simulink library "Library_Steering"  (R2023a)
settings: Solver=VariableStepAuto  StartTime=0.0  StopTime=10.0  RelTol=1e-3
undefined symbols (not defined in the file or in its folder): SteeringLeft, SteeringRight
libraries: mbd_s32k1xx_ec_toolbox x17, simulink x8, $bdroot x3
(part 2 of 2)

== stateflow chart Library_Steering/Steering_Mgmt_FSM/Chart ==
  state CAN_Watchdog [parallel]
    entry:
    lastCANWatchDogTime = 0;
    settings: executionOrder=2
    state CAN_Good
    state CAN_Lost
    (default) -> CAN_Good
    CAN_Good -> CAN_Watchdog [order 2] : [input_CAN_timeStamp > lastCANWatchDogTime]{lastCANWatchDogTime = input_CAN_timeStamp}
    CAN_Good -> CAN_Lost [order 1] : [elapsed > param_CANTimeOut & lastCANWatchDogTime ~= 0]{send(CAN_WD_Timeout,Steering_Mode)}
    CAN_Lost -> CAN_Good : FAULT_RESET
  state Steering_Mode [parallel]
    % ALL SDO TRANSFERS MUST BE MADE IN THIS STATE AND NOWHERE ELSE TO AVOID CONFLICTS
    settings: executionOrder=4
    state Steering_Degraded
      entry:
      output_chart_state = 2;
      state SetCaptureMode
        entry:
        output_chart_substate = uint8(hex2dec('21'));
        % Shut off SDO output enable
        output_SDO_enable = 0;
        exit:
        % Shut off SDO output upon exiting this state
        output_SDO_enable = 0;
        state SDOSend
          entry:
          output_SDO_enable = 0;
          output_SDO_data = cast([hex2dec('2B'); hex2dec('00'); hex2dec('24'); 0; hex2dec('45'); hex2dec('05'); 0; 0;],'uint8');
          output_SDO_enable = 1;
        state SDOWait1
          entry:
          output_SDO_enable = 0;
          output_SDO_data = cast([hex2dec('40'); hex2dec('00'); hex2dec('24'); 0; 0; 0; 0; 0],'uint8');
          output_SDO_enable = 1;
        state SDOWait2
          entry:
          output_SDO_enable = 0;
        (default) -> Steering_Mode.Steering_Degraded.SetCaptureMode.SDOSend
        Steering_Mode.Steering_Degraded.SetCaptureMode.SDOSend -> Steering_Mode.Steering_Degraded.SetCaptureMode.SDOWait1 : [input_SDOBuffer == 0]
        Steering_Mode.Steering_Degraded.SetCaptureMode.SDOWait2 -> Steering_Mode.Steering_Degraded.SetCaptureMode.SDOSend : [elapsed > 0.5 && input_SDOBuffer == 0]
        Steering_Mode.Steering_Degraded.SetCaptureMode.SDOWait1 -> Steering_Mode.Steering_Degraded.SetCaptureMode.SDOWait2 : [input_SDOBuffer == 0]
      state SetVelocityLimit
        entry:
        output_chart_substate = uint8(hex2dec('22'));
        % Shut off SDO output enable
        output_SDO_enable = 0;
        exit:
        % Shut off SDO output upon exiting this state
        output_SDO_enable = 0;
        state SDOSend
          entry:
          output_SDO_enable = 0;
          output_SDO_data = cast([hex2dec('23'); hex2dec('80'); hex2dec('60'); 0; 32; 3; 0; 0;],'uint8');
          output_SDO_enable = 1;
        state SDOWait1
          entry:
          output_SDO_enable = 0;
          output_SDO_data = cast([hex2dec('40'); hex2dec('80'); hex2dec('60'); 0; 0; 0; 0; 0],'uint8');
          output_SDO_enable = 1;
        state SDOWait2
          entry:
          output_SDO_enable = 0;
        (default) -> Steering_Mode.Steering_Degraded.SetVelocityLimit.SDOSend
        Steering_Mode.Steering_Degraded.SetVelocityLimit.SDOSend -> Steering_Mode.Steering_Degraded.SetVelocityLimit.SDOWait1 : [input_SDOBuffer == 0]
        Steering_Mode.Steering_Degraded.SetVelocityLimit.SDOWait2 -> Steering_Mode.Steering_Degraded.SetVelocityLimit.SDOSend : [elapsed > 0.5 && input_SDOBuffer == 0]
        Steering_Mode.Steering_Degraded.SetVelocityLimit.SDOWait1 -> Steering_Mode.Steering_Degraded.SetVelocityLimit.SDOWait2 : [input_SDOBuffer == 0]
      state SetCSPMode
        entry:
        output_chart_substate = uint8(hex2dec('23'));
        % Shut off SDO output enable
        output_SDO_enable = 0;
        exit:
        % Shut off SDO output upon exiting this state
        output_SDO_enable = 0;
        state SDOSend
          entry:
          output_SDO_enable = 0;
          output_SDO_data = cast([hex2dec('2F'); hex2dec('60'); hex2dec('60'); 0; 8; 0; 0; 0;],'uint8');
          output_SDO_enable = 1;
        state SDOWait1
          entry:
          output_SDO_enable = 0;
          output_SDO_data = cast([hex2dec('40'); hex2dec('60'); hex2dec('60'); 0; 0; 0; 0; 0],'uint8');
          output_SDO_enable = 1;
        state SDOWait2
          entry:
          output_SDO_enable = 0;
        (default) -> Steering_Mode.Steering_Degraded.SetCSPMode.SDOSend
        Steering_Mode.Steering_Degraded.SetCSPMode.SDOSend -> Steering_Mode.Steering_Degraded.SetCSPMode.SDOWait1 : [input_SDOBuffer == 0]
        Steering_Mode.Steering_Degraded.SetCSPMode.SDOWait2 -> Steering_Mode.Steering_Degraded.SetCSPMode.SDOSend : [elapsed > 0.5 && input_SDOBuffer == 0]
        Steering_Mode.Steering_Degraded.SetCSPMode.SDOWait1 -> Steering_Mode.Steering_Degraded.SetCSPMode.SDOWait2 : [input_SDOBuffer == 0]
      state CheckForCaptures
        entry:
        output_chart_substate = uint8(hex2dec('24'));
        % Shut off SDO output enable
        output_SDO_enable = 0;
        % Enable transmission for the position target PDO
        output_PDO_enable = 1;
        exit:
        output_SDO_enable = 0;
        state SDOSend
          entry:
          output_SDO_enable = 0;
          output_SDO_data = cast([hex2dec('40'); hex2dec('01'); hex2dec('24'); 0; 0; 0; 0; 0;],'uint8');
          output_SDO_enable = 1;
        state SDOWait2
          entry:
          output_SDO_enable = 0;
        (default) -> Steering_Mode.Steering_Degraded.CheckForCaptures.SDOSend
        Steering_Mode.Steering_Degraded.CheckForCaptures.SDOSend -> Steering_Mode.Steering_Degraded.CheckForCaptures.SDOWait2
        Steering_Mode.Steering_Degraded.CheckForCaptures.SDOWait2 -> Steering_Mode.Steering_Degraded.CheckForCaptures.SDOSend : [input_SDOBuffer == 0]
      state FinalCalibration
        output_chart_substate = uint8(hex2dec('25'));
        % Shut off SDO output enable
        output_SDO_enable = 0;
        % Keep the PDO enabled for the position setpoint update
        output_PDO_enable = 1;
        exit:
        % Shut off SDO output upon exiting this state
        output_SDO_enable = 0;
        output_PDO_enable = 1;
        state RequestIndexPos
          entry:
          output_SDO_enable = 0;
          output_SDO_data = cast([hex2dec('40'); hex2dec('02'); hex2dec('24'); 0; 0; 0; 0; 0;],'uint8');
          output_SDO_enable = 1;
        state RequestHomePos
          entry:
          output_SDO_enable = 0;
          output_SDO_data = cast([hex2dec('40'); hex2dec('03'); hex2dec('24'); 0; 0; 0; 0; 0;],'uint8');
          output_SDO_enable = 1;
        state RequestHighSpeedCapturePos
          entry:
          output_SDO_enable = 0;
          output_SDO_data = cast([hex2dec('40'); hex2dec('05'); hex2dec('24'); 0; 0; 0; 0; 0;],'uint8');
          output_SDO_enable = 1;
        state WaitForIndexPos
          entry:
          output_SDO_enable = 0;
        state WaitForHomePos1
          entry:
          output_SDO_enable = 0;
        state WaitForHighSpeedCapturePos
          entry:
          output_SDO_enable = 0;
        state StoreIndex
          entry:
          output_SDO_enable = 0;
          index_position = SDO2Integer32(input_SDO_message);
        state StoreHome
          entry:
          output_SDO_enable = 0;
          home_position = SDO2Integer32(input_SDO_message);
        state StoreHighSpeedCapturePos
          entry:
          output_SDO_enable = 0;
          highspeed_position = SDO2Integer32(input_SDO_message);
        state CalculateZeroOffset
          entry:
          output_SDO_enable = 0;
          hall_width = highspeed_position - home_position;
          int_offset_2 = floor((highspeed_position - index_position)/(4000));
          int_offset_1 = floor((home_position - index_position)/(4000));
          home_index = index_position + 4000*max(int_offset_1,int_offset_2);
          home_offset = min(home_position - home_index,highspeed_position - home_index);
          final_offset = home_index;
        (default) -> RequestIndexPos
        StoreIndex -> RequestHomePos : [input_SDOBuffer == 0]
        StoreHome -> RequestHighSpeedCapturePos : [input_SDOBuffer == 0]
        RequestIndexPos -> WaitForIndexPos : [input_SDOBuffer == 0]
        WaitForIndexPos -> RequestIndexPos [order 2] : [elapsed > 0.5 && input_SDOBuffer == 0]
        RequestHomePos -> WaitForHomePos1 : [input_SDOBuffer == 0]
        WaitForHomePos1 -> RequestHomePos [order 2] : [elapsed > 0.5 && input_SDOBuffer == 0]
        RequestHighSpeedCapturePos -> WaitForHighSpeedCapturePos : [input_SDOBuffer == 0]
        WaitForHighSpeedCapturePos -> RequestHighSpeedCapturePos [order 2] : [elapsed > 0.5 && input_SDOBuffer == 0]
        WaitForIndexPos -> StoreIndex [order 1] : [input_SDO_message(2) == hex2dec('02') && input_SDO_message(3) == hex2dec('24')]
        WaitForHomePos1 -> StoreHome [order 1] : [input_SDO_message(2) == hex2dec('03') && input_SDO_message(3) == hex2dec('24')]
        WaitForHighSpeedCapturePos -> StoreHighSpeedCapturePos [order 1] : [input_SDO_message(2) == hex2dec('05') && input_SDO_message(3) == hex2dec('24')]
        StoreHighSpeedCapturePos -> CalculateZeroOffset
      state SetOffset
        % Set Index 0x607C with a new value to adjust the zero position of the steering system relative to the arbitary home that was set at startup
        entry:
        final_offset = final_offset + param_finalOffsetAlignment;
        output_chart_substate = uint8(hex2dec('26'));
        output_PDO_enable = 1;
        output_position_offset = 0;
        offset_bytes = [0; 0; 0; 0];
        offset_bytes(1) = extractByte(output_position_offset,1);
        offset_bytes(2) = extractByte(output_position_offset,2);
        offset_bytes(3) = extractByte(output_position_offset,3);
        offset_bytes(4) = extractByte(output_position_offset,4);
        state SDOSend
          entry:
          offset_bytes(1) = extractByte(output_position_offset,1);
          offset_bytes(2) = extractByte(output_position_offset,2);
          offset_bytes(3) = extractByte(output_position_offset,3);
          offset_bytes(4) = extractByte(output_position_offset,4);
          output_SDO_enable = 0;
          output_SDO_data = cast([hex2dec('23'); hex2dec('B0'); hex2dec('60'); 0; offset_bytes],'uint8');
          output_SDO_enable = 1;
        state SDOWait1
          entry:
          output_SDO_enable = 0;
          output_SDO_data = cast([hex2dec('40'); hex2dec('B0'); hex2dec('60'); 0; 0; 0; 0; 0],'uint8');
          output_SDO_enable = 1;
        state SDOWait2
          entry:
          output_SDO_enable = 0;
        (default) -> Steering_Mode.Steering_Degraded.SetOffset.SDOSend
        Steering_Mode.Steering_Degraded.SetOffset.SDOWait2 -> Steering_Mode.Steering_Degraded.SetOffset.SDOSend : [elapsed > 0.02 && input_SDOBuffer == 0]{output_position_offset = sign(final_offset)*min(abs(output_position_offset)+...
            | param_alignmentSlewRate,abs(final_offset));}
        Steering_Mode.Steering_Degraded.SetOffset.SDOSend -> Steering_Mode.Steering_Degraded.SetOffset.SDOWait1 : [input_SDOBuffer == 0]
        Steering_Mode.Steering_Degraded.SetOffset.SDOWait1 -> Steering_Mode.Steering_Degraded.SetOffset.SDOWait2 : [all(input_SDO_message(2:8) == cast([hex2dec('B0');...
            |  hex2dec('60'); 0; offset_bytes],'uint8'))]
      state SetVelocityLimit1
        entry:
        output_chart_substate = uint8(hex2dec('27'));
        % Shut off SDO output enable
        output_SDO_enable = 0;
        exit:
        % Shut off SDO output upon exiting this state
        output_SDO_enable = 0;
        state SDOSend
          entry:
          output_SDO_enable = 0;
          output_SDO_data = cast([hex2dec('23'); hex2dec('80'); hex2dec('60'); 0; 255; 79; 0; 0;],'uint8');
          output_SDO_enable = 1;
        state SDOWait1
          entry:
          output_SDO_enable = 0;
          output_SDO_data = cast([hex2dec('40'); hex2dec('80'); hex2dec('60'); 0; 0; 0; 0; 0],'uint8');
          output_SDO_enable = 1;
        state SDOWait2
          entry:
          output_SDO_enable = 0;
        (default) -> Steering_Mode.Steering_Degraded.SetVelocityLimit1.SDOSend
        Steering_Mode.Steering_Degraded.SetVelocityLimit1.SDOSend -> Steering_Mode.Steering_Degraded.SetVelocityLimit1.SDOWait1 : [input_SDOBuffer == 0]
        Steering_Mode.Steering_Degraded.SetVelocityLimit1.SDOWait2 -> Steering_Mode.Steering_Degraded.SetVelocityLimit1.SDOSend : [elapsed > 0.5 && input_SDOBuffer == 0]
        Steering_Mode.Steering_Degraded.SetVelocityLimit1.SDOWait1 -> Steering_Mode.Steering_Degraded.SetVelocityLimit1.SDOWait2 : [input_SDOBuffer == 0]
      (default) -> SetCaptureMode
      SetCaptureMode -> SetVelocityLimit : [all(input_SDO_message == cast([hex2dec('4B'); hex2dec('00'); hex2dec('24'); 0; hex2dec('45'); hex2dec('05'); 0; 0;],'uint8'))]
      SetVelocityLimit -> SetCSPMode : [all(input_SDO_message == cast([hex2dec('43'); hex2dec('80'); hex2dec('60'); 0; 32; 3; 0; 0;],'uint8'))]
      SetCSPMode -> CheckForCaptures : [all(input_SDO_message == cast([hex2dec('4F'); hex2dec('60'); hex2dec('60'); 0; 8; 0; 0; 0;],'uint8'))]
      CalculateZeroOffset -> CheckForCaptures [order 2]
      CheckForCaptures -> FinalCalibration : [input_SDO_message(2) == hex2dec('01') &&...
          |  input_SDO_message(3) == hex2dec('24') &&...
          |  bitand(uint8(hex2dec('11')),input_SDO_message(5)) == uint8(hex2dec('11')) &&...
          |  bitand(uint8(hex2dec('01')),input_SDO_message(6)) == uint8(hex2dec('01'))]
      CalculateZeroOffset -> SetOffset [order 1] : [final_offset < param_finalOffsetHighThresh && final_offset > param_finalOffsetLowThresh && ...
          | [hall_width > param_hallWidthLowThresh && hall_width < param_hallWidthHighThresh && ...
          | home_offset > param_homeOffsetLowThresh && home_offset < param_homeOffsetHighThresh && ...
          | int_offset_1 - int_offset_2 < param_intOffsetThresh && int_offset_2 - int_offset_1 < param_intOffsetThresh]]
      SetOffset -> SetVelocityLimit1 : [output_position_offset == final_offset]
    state Steering_Operational
      entry:
      output_chart_state = 3
      output_chart_substate = uint8(hex2dec('30'));
      output_PDO_enable = 1;
      output_SDO_data = cast([hex2dec('40');...
      hex2dec('41'); hex2dec('60'); hex2dec('00');...
      hex2dec('00'); hex2dec('00'); hex2dec('00');...
      hex2dec('00')],'uint8');
      output_SDO_enable = 1;
      output_actual_position = SDO2Integer32(input_SDO_message);
    state Steering_Startup
      entry:
      output_chart_state = 1;
      state ConfirmNMTUp  % Sends NMT (network management) message to start up the CANOpen node being controlled
        % Actions to perform once upon entering this state
        entry:
        % Set chart state indicator variable
        output_chart_substate = uint8(hex2dec('11'));
        % Actions to perform once when exiting this state
        exit:
        % Disable the NMT message send output port when done
        output_NMT_enable = 0;
        output_SDO_enable = 0;
        state NMTQuerySend  % Send the NMT query message via SDO format
          entry:
          % Set the SDO data packet to request the device network status word (0x21B4)
          output_SDO_data = cast([hex2dec('40'); hex2dec('B4'); ...
          hex2dec('21'); hex2dec('00'); hex2dec('00');...
          hex2dec('00'); hex2dec('00'); hex2dec('00')],'uint8');
          % Enable the SDO send
          output_SDO_enable = 1;
        state SDOWait  % Wait to send next SDO message
          entry:
          output_NMT_enable = 0;
        state NMTSetActive % Enable the block that sends the NMT active message
          entry:
          % Enable the NMT send
          output_NMT_enable = 1;
        state NMTWait  % Wait to send next NMT message
          entry:
          output_SDO_enable = 0;
        (default) -> Steering_Mode.Steering_Startup.ConfirmNMTUp.SDOWait  % Wait to send next SDO message
        Steering_Mode.Steering_Startup.ConfirmNMTUp.SDOWait  % Wait to send next SDO message -> Steering_Mode.Steering_Startup.ConfirmNMTUp.NMTQuerySend  % Send the NMT query message via SDO format : [input_SDOBuffer == 0]
        Steering_Mode.Steering_Startup.ConfirmNMTUp.NMTSetActive % Enable the block that sends the NMT active message -> Steering_Mode.Steering_Startup.ConfirmNMTUp.SDOWait  % Wait to send next SDO message
        Steering_Mode.Steering_Startup.ConfirmNMTUp.NMTQuerySend  % Send the NMT query message via SDO format -> Steering_Mode.Steering_Startup.ConfirmNMTUp.NMTWait  % Wait to send next NMT message
        Steering_Mode.Steering_Startup.ConfirmNMTUp.NMTWait  % Wait to send next NMT message -> Steering_Mode.Steering_Startup.ConfirmNMTUp.NMTSetActive % Enable the block that sends the NMT active message : [input_NMTBuffer == 0]
      state CheckEnableAmpStatus  % Sends SDO message until the amp status message shows that it is enabled
        % Actions to perform once upon entering this state
        entry:
        % Set chart state indicator variable
        output_chart_substate = uint8(hex2dec('12'));
        state StatusQuerySend  % Send the amp status query message via SDO format
          entry:
          % Set the SDO data packet to request the amp status word (0x6041)
          output_SDO_data = cast([hex2dec('40'); hex2dec('41'); ...
          hex2dec('60'); hex2dec('00'); hex2dec('00');...
          hex2dec('00'); hex2dec('00'); hex2dec('00')],'uint8');
          % Enable the SDO send
          output_SDO_enable = 1;
        state SDOWait  % Wait to send next SDO message
          entry:
          output_SDO_enable = 0;
        state SetAmpEnabled % Enable the block that sends the amp enable message
          entry:
          % Set the SDO data packet to set the amp control word (0x6040)
          output_SDO_data = cast([hex2dec('2B'); hex2dec('40'); ...
          hex2dec('60'); hex2dec('00'); hex2dec('07');...
          hex2dec('00'); hex2dec('00'); hex2dec('00')],'uint8');
          % Enable the SDO send
          output_SDO_enable = 1;
        state SDOWait1  % Wait to send next NMT message
          entry:
          output_SDO_enable = 0;
        (default) -> Steering_Mode.Steering_Startup.CheckEnableAmpStatus.SDOWait  % Wait to send next SDO message
        Steering_Mode.Steering_Startup.CheckEnableAmpStatus.SDOWait  % Wait to send next SDO message -> Steering_Mode.Steering_Startup.CheckEnableAmpStatus.StatusQuerySend  % Send the amp status query message via SDO format : [input_SDOBuffer == 0]
        Steering_Mode.Steering_Startup.CheckEnableAmpStatus.SetAmpEnabled % Enable the block that sends the amp enable message -> Steering_Mode.Steering_Startup.CheckEnableAmpStatus.SDOWait  % Wait to send next SDO message
        Steering_Mode.Steering_Startup.CheckEnableAmpStatus.StatusQuerySend  % Send the amp status query message via SDO format -> Steering_Mode.Steering_Startup.CheckEnableAmpStatus.SDOWait1  % Wait to send next NMT message
        Steering_Mode.Steering_Startup.CheckEnableAmpStatus.SDOWait1  % Wait to send next NMT message -> Steering_Mode.Steering_Startup.CheckEnableAmpStatus.SetAmpEnabled % Enable the block that sends the amp enable message : [input_SDOBuffer == 0]
      state CheckOperatingMode  % Sends SDO message until the operating mode is determined, and sends the state machine either to finish startup or resuming operation
        % Actions to perform once upon entering this state
        entry:
        % Set chart state indicator variable
        output_chart_substate = uint8(hex2dec('13'));
        state SDOWait1  % Wait to send next SDO message
          entry:
          output_SDO_enable = 0;
        state ModeQuerySend  % Send the amp status query message via SDO format
          entry:
          % Set the SDO data packet to request the amp status word (0x6041)
          output_SDO_data = cast([hex2dec('40'); hex2dec('61'); ...
          hex2dec('60'); hex2dec('00'); hex2dec('00');...
          hex2dec('00'); hex2dec('00'); hex2dec('00')],'uint8');
          % Enable the SDO send
          output_SDO_enable = 1;
        (default) -> SDOWait1  % Wait to send next SDO message
        SDOWait1  % Wait to send next SDO message -> ModeQuerySend  % Send the amp status query message via SDO format : [input_SDOBuffer == 0]
        ModeQuerySend  % Send the amp status query message via SDO format -> SDOWait1  % Wait to send next SDO message
      state CollectAnalogValues  % Controls acquisition of desired number of analog measurements until an average can be generated
        % Actions to perform once upon entering this state
        entry:
        % Set chart state indicator variable to 0x14
        output_chart_substate = uint8(hex2dec('14'));
        % Initialize a counter for the number of measurements collected
        meas_counter = 0;
        % Initialize a running sum variable to zero
        running_mean = 0;
        % Initialize the running standard deviation variable to zero
        running_std = 0;
        % Initialize a variable to keep track of the time stamp of the most recent SDO message received
        % to avoid duplicating measurements in the average
        prevTime = input_CAN_timeStamp;
        % Set the SDO transmit message to request the analog measurement object
        output_SDO_data = cast([hex2dec('40'); hex2dec('00'); hex2dec('22'); hex2dec('00'); hex2dec('00');...
        hex2dec('00'); hex2dec('00'); hex2dec('00')],'uint8');
        % Enable SDO output transmission (holding this high will send continuously)
        output_SDO_enable = 1;
        % Actions to perform once per cycle
        during:
        % Check for a new SDO message with the analog measurement value. If a new measurement is available, average it
        receiveAnalogInput;
        % Exit condition is that 50 measurements have been averaged together
      state receiveAnalogInput [function]
        (default) -> (junction 364) : {potVoltage = SDO2Integer16(input_SDO_message)}
        (junction 364) -> (junction 365) [order 1] : [potVoltage > param_minPotAvgVal && potVoltage < param_maxPotAvgVal && meas_counter <= param_initNumPotReadings &&...
            |  input_CAN_timeStamp ~= prevTime && input_SDO_message(2) == hex2dec('00') && input_SDO_message(3) == hex2dec('22')]
        (junction 364) -> (junction 366) [order 2]
        (junction 365) -> (junction 367) : {meas_counter = meas_counter + 1;
            |  residual = (cast(potVoltage,'double') - running_mean);
            |  running_mean = running_mean + residual/meas_counter;
            |  running_std = running_std + (residual*(cast(potVoltage,'double') - running_mean) - running_std)/meas_counter;
            |  prevTime = input_CAN_timeStamp;}
        (junction 367) -> (junction 366)
      state WriteHomePos  % Convert the raw analog values to encoder counts and set the motor position object on the amp
        % Actions to perform once upon entering this state
        entry:
        % Set chart state indicator variable to 0x15
        output_chart_substate = uint8(hex2dec('15'));
        % Disable transmission of the SDO message until the message data bytes are updated
        output_SDO_enable = 0;
        % Convert the potentiometer position to encoder counts
        output_actual_position = cast(param_potEncSlope*running_mean + param_potEncInt,'int32');
        pos_encoder_bytes = [0; 0; 0; 0];
        pos_encoder_bytes(1) = extractByte(output_actual_position,1);
        pos_encoder_bytes(2) = extractByte(output_actual_position,2);
        pos_encoder_bytes(3) = extractByte(output_actual_position,3);
        pos_encoder_bytes(4) = extractByte(output_actual_position,4);
        % Set the SDO message data that should be echoed back to move to the next state
        Position_Written_Expected_Bytes = [hex2dec('43'); hex2dec('63'); hex2dec('60'); hex2dec('00'); pos_encoder_bytes];
        exit:
        % Shut off SDO output upon exiting this state
        output_SDO_enable = 0;
        state SDOSend
          entry:
          output_SDO_enable = 0;
          output_SDO_data = cast([hex2dec('23'); hex2dec('63'); hex2dec('60'); hex2dec('00'); pos_encoder_bytes],'uint8');
          output_SDO_enable = 1;
        state SDOWait1
          entry:
          output_SDO_enable = 0;
          output_SDO_data = cast([hex2dec('40'); hex2dec('63'); hex2dec('60'); 0; 0; 0; 0; 0],'uint8');
          output_SDO_enable = 1;
        state SDOWait2
          entry:
          output_SDO_enable = 0;
        (default) -> Steering_Mode.Steering_Startup.WriteHomePos.SDOSend
        Steering_Mode.Steering_Startup.WriteHomePos.SDOSend -> Steering_Mode.Steering_Startup.WriteHomePos.SDOWait1 : [input_SDOBuffer == 0]
        Steering_Mode.Steering_Startup.WriteHomePos.SDOWait2 -> Steering_Mode.Steering_Startup.WriteHomePos.SDOSend : [elapsed > 0.5 && input_SDOBuffer == 0]
        Steering_Mode.Steering_Startup.WriteHomePos.SDOWait1 -> Steering_Mode.Steering_Startup.WriteHomePos.SDOWait2 : [input_SDOBuffer == 0]
      (default) -> Steering_Mode.Steering_Startup.ConfirmNMTUp  % Sends NMT (network management) message to start up the CANOpen node being controlled
      Steering_Mode.Steering_Startup.ConfirmNMTUp  % Sends NMT (network management) message to start up the CANOpen node being controlled -> Steering_Mode.Steering_Startup.CheckEnableAmpStatus  % Sends SDO message until the amp status message shows that it is enabled : [input_SDO_message(2) == cast(hex2dec('B4'),'uint8') && input_SDO_message(3) == cast(hex2dec('21'),'uint8') && bitand(input_SDO_message(5),cast(hex2dec('03'),'uint8')) == cast(3,'uint8')]
      Steering_Mode.Steering_Startup.CheckEnableAmpStatus  % Sends SDO message until the amp status message shows that it is enabled -> CheckOperatingMode  % Sends SDO message until the operating mode is determined, and sends the state machine either to finish startup or resuming operation : [input_SDO_message(2) == cast(hex2dec('41'),'uint8') && input_SDO_message(3) == cast(hex2dec('60'),'uint8') && bitand(input_SDO_message(5),cast(hex2dec('33'),'uint8')) == cast(hex2dec('33'),'uint8')]
      CheckOperatingMode  % Sends SDO message until the operating mode is determined, and sends the state machine either to finish startup or resuming operation -> CollectAnalogValues  % Controls acquisition of desired number of analog measurements until an average can be generated [order 2] : [input_SDO_message(2) == cast(hex2dec('61'),'uint8') && input_SDO_message(3) == cast(hex2dec('60'),'uint8')]
      CollectAnalogValues  % Controls acquisition of desired number of analog measurements until an average can be generated -> (junction 613) : [meas_counter >...
          |  param_initNumPotReadings]
      (junction 613) -> CollectAnalogValues  % Controls acquisition of desired number of analog measurements until an average can be generated [order 2]
      (junction 613) -> WriteHomePos  % Convert the raw analog values to encoder counts and set the motor position object on the amp [order 1] : [running_mean > param_minPotAvgVal && running_mean < param_maxPotAvgVal && running_std < param_maxPotSTD]
    state Steering_Fault
      entry:
      output_chart_substate = uint8(hex2dec('00'));
      output_PDO_enable = 0;
      output_chart_state = 0;
      output_SDO_data = cast([hex2dec('2B');...
      hex2dec('40'); hex2dec('60'); hex2dec('00');...
      hex2dec('05'); hex2dec('00'); hex2dec('00');...
      hex2dec('00')],'uint8');
      output_SDO_enable = 1;
    Steering_Degraded -> Steering_Fault [commented out] : AMP_FAULT
    Steering_Degraded -> Steering_Fault : CAN_WD_Timeout
    Steering_Operational -> Steering_Fault [commented out] : AMP_FAULT
    Steering_Operational -> Steering_Fault : CAN_WD_Timeout
    (default) -> Steering_Startup
    Steering_Startup -> Steering_Fault [order 1] : CAN_WD_Timeout
    Steering_Startup -> Steering_Fault [commented out] : AMP_FAULT
    Steering_Startup -> Steering_Fault [order 2] : [elapsed > param_startupTimeOut]...
        | {startup_timeout = 10}
    Steering_Fault -> Steering_Startup : FAULT_RESET
    CheckOperatingMode  % Sends SDO message until the operating mode is determined, and sends the state machine either to finish startup or resuming operation -> Steering_Degraded [order 1] : [input_SDO_message(2) == cast(hex2dec('61'),'uint8')...
        |  && input_SDO_message(3) == cast(hex2dec('60'),'uint8')...
        |  && input_SDO_message(5) == uint8(8)]
    SetVelocityLimit1 -> Steering_Operational : [all(input_SDO_message == cast([hex2dec('43'); hex2dec('80'); hex2dec('60'); 0; 255; 79; 0; 0;],'uint8'))]
    WriteHomePos  % Convert the raw analog values to encoder counts and set the motor position object on the amp -> Steering_Degraded : [all(input_SDO_message == Position_Written_Expected_Bytes)]
  state Fault_Lamp_Control [parallel]
    settings: executionOrder=1
    state Steady_OFF
      during:
      output_fault_lamp = 0;
    state Blink_OFF
      during:
      output_fault_lamp = 0;
    state Blink_ON
      during:
      output_fault_lamp = 1;
    state Steady_ON
      during:
      output_fault_lamp = 1;
    Steady_OFF -> Fault_Lamp_Control : [output_chart_state ~= 3]
    (junction 517) -> Steady_OFF [order 2] : [output_chart_state == 3]
    Blink_ON -> Steady_OFF [order 1] : [output_chart_state == 3]
    Blink_OFF -> Steady_OFF [order 1] : [output_chart_state == 3]
    Blink_OFF -> Blink_ON [order 3] : [elapsed > output_chart_state*0.2]
    (default) -> (junction 517)
    (junction 517) -> Blink_ON [order 3]
    (junction 517) -> Steady_ON [order 1] : [output_chart_state == 0]
    Blink_ON -> Blink_OFF [order 3] : [elapsed > output_chart_state*0.2]
    Blink_ON -> Steady_ON [order 2] : [output_chart_state == 0]
    Blink_OFF -> Steady_ON [order 2] : [output_chart_state == 0]
    Steady_ON -> Fault_Lamp_Control : [output_chart_state ~= 0]
  state Steering_Fault_Detection [parallel]
    settings: executionOrder=3
    state No_Fault
    state Faulted
      entry:
      send(AMP_FAULT,Steering_Mode)
      state ConfirmNMTUp  % Sends NMT (network management) message to start up the CANOpen node being controlled
        % Actions to perform once upon entering this state
        entry:
        % Set chart state indicator variable
        output_chart_substate = uint8(hex2dec('11'));
        % Actions to perform once when exiting this state
        exit:
        % Disable the NMT message send output port when done
        output_NMT_enable = 0;
        output_SDO_enable = 0;
        state NMTQuerySend  % Send the NMT query message via SDO format
          entry:
          % Set the SDO data packet to request the device network status word (0x21B4)
          output_SDO_data = cast([hex2dec('40'); hex2dec('B4'); ...
          hex2dec('21'); hex2dec('00'); hex2dec('00');...
          hex2dec('00'); hex2dec('00'); hex2dec('00')],'uint8');
          % Enable the SDO send
          output_SDO_enable = 1;
        state SDOWait  % Wait to send next SDO message
          entry:
          output_NMT_enable = 0;
        state NMTSetActive % Enable the block that sends the NMT active message
          entry:
          % Enable the NMT send
          output_NMT_enable = 1;
        state NMTWait  % Wait to send next NMT message
          entry:
          output_SDO_enable = 0;
        (default) -> Steering_Fault_Detection.Faulted.ConfirmNMTUp.SDOWait  % Wait to send next SDO message
        Steering_Fault_Detection.Faulted.ConfirmNMTUp.SDOWait  % Wait to send next SDO message -> Steering_Fault_Detection.Faulted.ConfirmNMTUp.NMTQuerySend  % Send the NMT query message via SDO format : [input_SDOBuffer == 0]
        Steering_Fault_Detection.Faulted.ConfirmNMTUp.NMTSetActive % Enable the block that sends the NMT active message -> Steering_Fault_Detection.Faulted.ConfirmNMTUp.SDOWait  % Wait to send next SDO message
        Steering_Fault_Detection.Faulted.ConfirmNMTUp.NMTQuerySend  % Send the NMT query message via SDO format -> Steering_Fault_Detection.Faulted.ConfirmNMTUp.NMTWait  % Wait to send next NMT message
        Steering_Fault_Detection.Faulted.ConfirmNMTUp.NMTWait  % Wait to send next NMT message -> Steering_Fault_Detection.Faulted.ConfirmNMTUp.NMTSetActive % Enable the block that sends the NMT active message : [input_NMTBuffer == 0]
      state CheckEnableAmpStatus  % Sends SDO message until the amp status message shows that it is enabled
        % Actions to perform once upon entering this state
        entry:
        % Set chart state indicator variable
        output_chart_substate = uint8(hex2dec('12'));
        state StatusQuerySend  % Send the amp status query message via SDO format
          entry:
          % Set the SDO data packet to request the amp status word (0x6041)
          output_SDO_data = cast([hex2dec('40'); hex2dec('41'); ...
          hex2dec('60'); hex2dec('00'); hex2dec('00');...
          hex2dec('00'); hex2dec('00'); hex2dec('00')],'uint8');
          % Enable the SDO send
          output_SDO_enable = 1;
        state SDOWait  % Wait to send next SDO message
          entry:
          output_SDO_enable = 0;
        state SetAmpEnabled % Enable the block that sends the amp enable message
          entry:
          % Set the SDO data packet to set the amp control word (0x6040)
          output_SDO_data = cast([hex2dec('2B'); hex2dec('40'); ...
          hex2dec('60'); hex2dec('00'); hex2dec('07');...
          hex2dec('00'); hex2dec('00'); hex2dec('00')],'uint8');
          % Enable the SDO send
          output_SDO_enable = 1;
        state SDOWait1  % Wait to send next NMT message
          entry:
          output_SDO_enable = 0;
        (default) -> Steering_Fault_Detection.Faulted.CheckEnableAmpStatus.SDOWait  % Wait to send next SDO message
        Steering_Fault_Detection.Faulted.CheckEnableAmpStatus.SDOWait  % Wait to send next SDO message -> Steering_Fault_Detection.Faulted.CheckEnableAmpStatus.StatusQuerySend  % Send the amp status query message via SDO format : [input_SDOBuffer == 0]
        Steering_Fault_Detection.Faulted.CheckEnableAmpStatus.SetAmpEnabled % Enable the block that sends the amp enable message -> Steering_Fault_Detection.Faulted.CheckEnableAmpStatus.SDOWait  % Wait to send next SDO message
        Steering_Fault_Detection.Faulted.CheckEnableAmpStatus.StatusQuerySend  % Send the amp status query message via SDO format -> Steering_Fault_Detection.Faulted.CheckEnableAmpStatus.SDOWait1  % Wait to send next NMT message
        Steering_Fault_Detection.Faulted.CheckEnableAmpStatus.SDOWait1  % Wait to send next NMT message -> Steering_Fault_Detection.Faulted.CheckEnableAmpStatus.SetAmpEnabled % Enable the block that sends the amp enable message : [input_SDOBuffer == 0]
      (default) -> Steering_Fault_Detection.Faulted.ConfirmNMTUp  % Sends NMT (network management) message to start up the CANOpen node being controlled
      Steering_Fault_Detection.Faulted.ConfirmNMTUp  % Sends NMT (network management) message to start up the CANOpen node being controlled -> Steering_Fault_Detection.Faulted.CheckEnableAmpStatus  % Sends SDO message until the amp status message shows that it is enabled : [input_SDO_message(2) == cast(hex2dec('B4'),'uint8') && input_SDO_message(3) == cast(hex2dec('21'),'uint8') && bitand(input_SDO_message(5),cast(hex2dec('03'),'uint8')) == cast(3,'uint8')]
    (default) -> No_Fault
    No_Fault -> Steering_Fault_Detection [order 1] : [bitand(input_amp_status_word(1),uint8(hex2dec('23'))) == uint8(hex2dec('23'))]
    No_Fault -> Faulted [order 2]
    Steering_Fault_Detection.Faulted.CheckEnableAmpStatus  % Sends SDO message until the amp status message shows that it is enabled -> No_Fault : [input_SDO_message(2) == cast(hex2dec('41'),'uint8') && input_SDO_message(3) == cast(hex2dec('60'),'uint8') ...
        | && bitand(input_SDO_message(5),cast(hex2dec('33'),'uint8')) == cast(hex2dec('33'),'uint8')]{send(FAULT_RESET)}
  data: inputVal function_input; byteNum function_input; outByte function_output; SDOMessageBytes function_input; returnInt16 function_output; inputVal function_input; byteNum function_input; outByte function_output; SDOMessageBytes function_input; returnInt32 function_output; output_NMT_enable output uint8 size=1; input_NMTBuffer input size=1; input_SDOBuffer input size=1; input_SDO_message input uint8 size=8; input_CAN_timeStamp input; meas_counter local double size=1; prevTime local; output_SDO_enable output; output_SDO_data output uint8 size=8; output_PDO_enable output; output_chart_state output; potVoltage local int16; Position_Written_Expected_Bytes local uint8 size=8; pos_encoder_bytes local uint8 size=4; home_position local int32 size=1; index_position local int32 size=1; output_chart_substate output uint8; output_fault_lamp output; running_mean local; running_std local; lastCANWatchDogTime local double; highspeed_position local int32 size=1; final_offset local int32; int_offset_1 local int32; hall_width local int32; int_offset_2 local int32; output_position_offset local int32; offset_bytes local uint8 size=4; home_index local int32; home_offset local int32; startup_timeout local =0; output_actual_position output; input_amp_status_word input uint8 size=2; param_CANTimeOut data_store_memory; param_initNumPotReadings data_store_memory; param_maxPotAvgVal data_store_memory; param_maxPotSTD data_store_memory; param_minPotAvgVal data_store_memory; param_potEncInt data_store_memory; param_potEncSlope data_store_memory; param_startupTimeOut data_store_memory; param_alignmentSlewRate data_store_memory; param_finalOffsetAlignment data_store_memory; param_finalOffsetHighThresh data_store_memory; param_finalOffsetLowThresh data_store_memory; param_hallWidthHighThresh data_store_memory; param_hallWidthLowThresh data_store_memory; param_homeOffsetHighThresh data_store_memory; param_homeOffsetLowThresh data_store_memory; param_intOffsetThresh data_store_memory
  events: CAN_WD_Timeout local FUNCTION_CALL_EVENT; AMP_FAULT local FUNCTION_CALL_EVENT; FAULT_RESET local FUNCTION_CALL_EVENT
  function outByte = extractByte(inputVal,byteNum):
    | function outByte = extractByte(inputVal,byteNum)
    | 
    | temp = typecast(inputVal,'uint8');
    | outByte = temp(byteNum);
  function returnInt16 = SDO2Integer16(SDOMessageBytes):
    | function returnInt16 = SDO2Integer16(SDOMessageBytes)
    | 
    | SDOIntegerBytes = cast(SDOMessageBytes,'uint16');
    | returnInt16 = cast(bitor(SDOIntegerBytes(5),...
    |     bitshift(SDOIntegerBytes(6),8)),'int16');
    | end
  function outByte = extractByte(inputVal,byteNum):
    | function outByte = extractByte(inputVal,byteNum)
    | 
    | temp = typecast(inputVal,'uint8');
    | outByte = temp(byteNum);
  function returnInt32 = SDO2Integer32(SDOMessageBytes):
    | function returnInt32 = SDO2Integer32(SDOMessageBytes)
    | 
    | SDOIntegerBytes = cast(SDOMessageBytes,'uint32');
    | returnInt32 = typecast(bitor(bitor(bitor(SDOIntegerBytes(5),...
    |     bitshift(SDOIntegerBytes(6),8)),...
    |     bitshift(SDOIntegerBytes(7),16)),...
    |     bitshift(SDOIntegerBytes(8),24)),...
    |     'int32');
    | returnInt32 = returnInt32(1);
    | end
